simulink model "smpld_data_sys_lb3"  (R2025b)
settings: Solver=ode45  StartTime=0.0  StopTime=20  FixedStep=T  MaxStep=0.01  RelTol=1e-12  AbsTol=1e-12  EnableMultiTasking=on
values from neighbouring files (symbols this model uses):
  K2 = 0.060911    [a7_new.m]
  K3 = -3.793    [a7_new.m]
libraries: cstblocks x3
settings Model: Creator=cnielsen  LastModifiedBy=hasan_khan
settings SolverCC: AutoScaleAbsTol=off  AlgebraicLoopSolver=TrustRegion
settings DataIOCC: SaveFormat=Array  SignalLoggingSaveFormat=ModelDataLogs  SaveOutput=off  SaveTime=off  ReturnWorkspaceOutputs=off  Refine=5
settings OptimizationCC: ExpressionDepthLimit=2147483647.0  LifeSpan=inf
settings DebuggingCC: UnderspecifiedInitializationDetection=Classic  MergeDetectMultiDrivingBlocksExec=none  SolverPrmCheckMsg=warning  FcnCallInpInsideContextMsg=warning  UnconnectedInputMsg=warning  UnconnectedOutputMsg=warning  UnconnectedLineMsg=warning  StateNameClashWarn=warning  SFUnexpectedBacktrackingDiag=warning  SFNoUnconditionalDefaultTransitionDiag=warning  SFExecutionAtInitializationDiag=none  ArithmeticOperatorsInVariantConditions=warning
settings HardwareCC: ProdBitPerPointer=32.0  ProdBitPerSizeT=32.0  ProdBitPerPtrDiffT=32.0  ProdLargestAtomicFloat=None  ProdIntDivRoundTo=Undefined  ProdEndianess=Unspecified  ProdWordSize=32.0  ProdHWDeviceType=32-bit Generic
settings ModelReferenceCC: PropagateSignalLabelsOutOfModel=off
settings SFSimCC: SimUseLocalCustomCode=off  CustomCodeUndefinedFunction=UseInterfaceOnly
settings RTWCC: RTWUseLocalCustomCode=off  GPUComputeCapability=3.5
settings CodeAppCC: StateflowObjectComments=on
settings GRTTargetCC: TargetLangStandard=C89/C90 (ANSI)  CombineOutputUpdateFcns=off  GRTInterface=on
settings ConfigComp: CovMetricSettings=dw  CovSaveCumulativeToWorkspaceVar=on  CovSaveSingleToWorkspaceVar=on  CovExternalEMLEnable=off
settings SimscapeCC: SimscapeLogDecimation=1  SimscapeLogDataHistory=5000

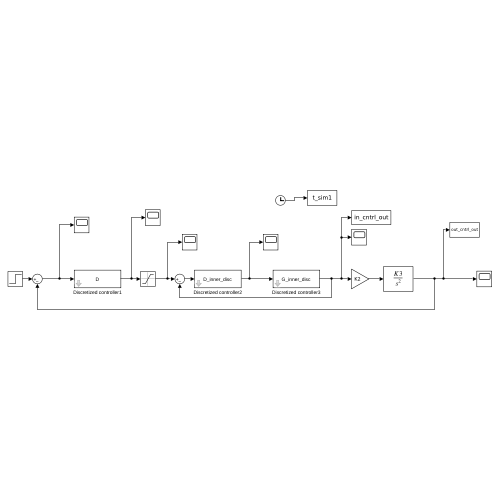
[thumbnail: Simulink's stored preview of the top-level diagram]
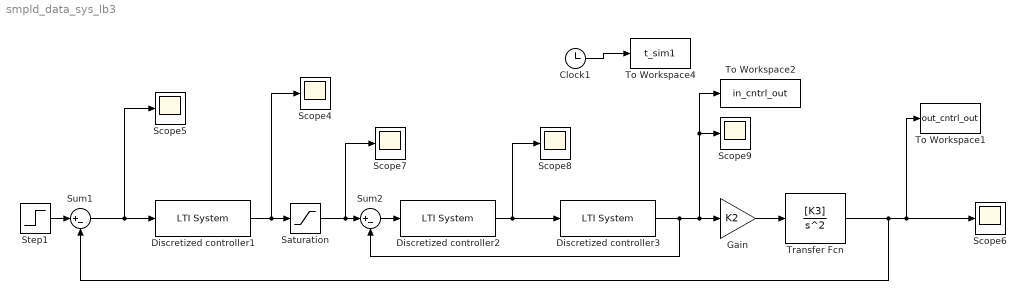
== system smpld_data_sys_lb3 ==
  Clock1 : Clock
  Discretized controller1 : cstblocks/LTI System  sys=D  IC=[]  PadeOrder=0
  Discretized controller2 : cstblocks/LTI System  sys=D_inner_disc  IC=[]  PadeOrder=0
  Discretized controller3 : cstblocks/LTI System  sys=G_inner_disc  IC=[]  PadeOrder=0
  Gain : Gain  Gain=K2
  Saturation : Saturate
  Scope{4..9} (6 alike) : Scope
      Scope4 settings: ActiveDisplayYMinimum=-7.94103  ActiveDisplayYMaximum=8.76404  DataLoggingVariableName=ScopeData3
      Scope5 settings: ActiveDisplayYMinimum=-7.94103  ActiveDisplayYMaximum=8.76404  DataLoggingVariableName=ScopeData4
      Scope6 settings: ActiveDisplayYMinimum=0.24996590680430081  ActiveDisplayYMaximum=1.6373414909323993  DataLoggingVariableName=ScopeData5
      Scope7 settings: ActiveDisplayYMinimum=-7.94103  ActiveDisplayYMaximum=8.76404  DataLoggingVariableName=ScopeData6
      Scope8 settings: ActiveDisplayYMinimum=-7.94103  ActiveDisplayYMaximum=8.76404  DataLoggingVariableName=ScopeData7
      Scope9 settings: ActiveDisplayYMinimum=-7.94103  ActiveDisplayYMaximum=8.76404  DataLoggingVariableName=ScopeData8
  Step1 : Step  Time=0  SampleTime=0.2764
  Sum1 : Sum  Inputs=|+-
  Sum2 : Sum  Inputs=|+-
  To Workspace1 : ToWorkspace  VariableName=out_cntrl_out  SampleTime=-1
  To Workspace2 : ToWorkspace  VariableName=in_cntrl_out  SampleTime=-1
  To Workspace4 : ToWorkspace  VariableName=t_sim1  SampleTime=-1
  Transfer Fcn : TransferFcn  Numerator=[K3]  Denominator=[1 0 0]
  wires:
  Step1/1 -> Sum1/1
  Transfer Fcn/1 -> To Workspace1/1, Scope6/1, Sum1/2
  Sum1/1 -> Discretized controller1/1, Scope5/1
  Discretized controller1/1 -> Scope4/1, Saturation/1
  Saturation/1 -> Scope7/1, Sum2/1
  Sum2/1 -> Discretized controller2/1
  Discretized controller2/1 -> Scope8/1, Discretized controller3/1
  Gain/1 -> Transfer Fcn/1
  Discretized controller3/1 -> To Workspace2/1, Scope9/1, Gain/1, Sum2/2
  Clock1/1 -> To Workspace4/1
